simulink model "L_vs_pos_tgt"  (R2021b)
settings: Solver=ode1  StartTime=0.0  StopTime=inf  FixedStep=1e-3  RelTol=1e-3  EnableMultiTasking=on
InitFcn:
  | voltage_gain = 1;
  | current_gain = 0.5*0.1;
libraries: speedgoatlib_IO102 x3, speedgoatlib_IO301 x2, slrealtimeutilitieslib x1, slrealtimeiplib x1
settings Model: sg_rtwmakecfg_data=_sglibc_  SimulationMode=external  Creator=tcraddoc  LastModifiedBy=wasynczu
settings SolverCC: ConcurrentTasks=on  AlgebraicLoopSolver=TrustRegion  PositivePriorityOrder=on
settings DataIOCC: SaveFormat=StructureWithTime  ReturnWorkspaceOutputs=off
settings OptimizationCC: BlockReduction=off  OptimizeBlockIOStorage=off  BufferReuse=off  GlobalBufferReuse=off  ExpressionFolding=off  LocalBlockOutputs=off
settings DebuggingCC: TasksWithSamePriorityMsg=none  SFMachineParentedDataDiag=warning  ArithmeticOperatorsInVariantConditions=warning
settings HardwareCC: ProdBitPerLong=64  ProdLongLongMode=on  ProdHWDeviceType=Intel->x86-64 (Linux 64)
settings SFSimCC: SimUseLocalCustomCode=off  CustomCodeUndefinedFunction=UseInterfaceOnly
settings RTWCC: Description=Simulink Real-Time  SystemTargetFile=slrealtime.tlc  TemplateMakefile=slrealtime_default_tmf  RTWUseLocalCustomCode=off  Toolchain=Simulink Real-Time Toolchain  BuildConfiguration=Faster Runs  CodeExecutionProfiling=on  TargetLang=C++
settings CodeAppCC: StateflowObjectComments=on

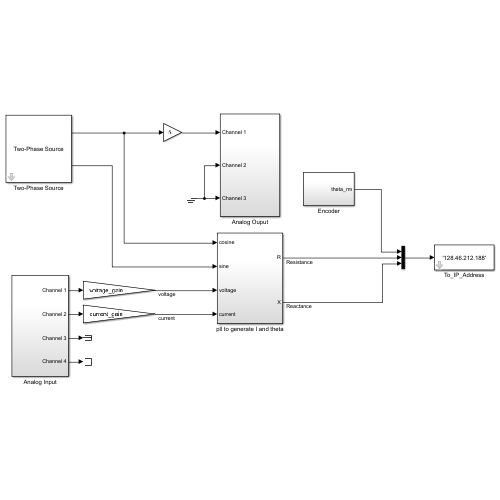
[thumbnail: Simulink's stored preview of the top-level diagram]
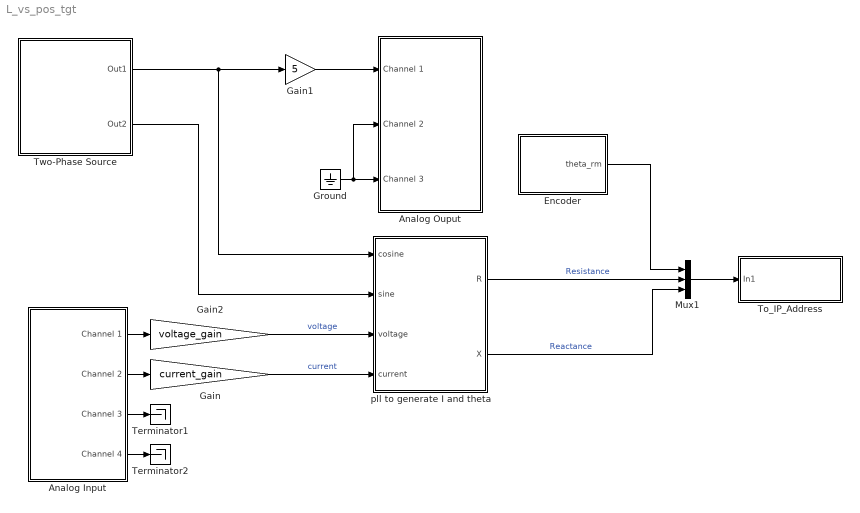
== system L_vs_pos_tgt ==
  Analog Input : Subsystem
  Analog Ouput : Subsystem
  Encoder : Subsystem
  Gain : Gain  Gain=current_gain
  Gain1 : Gain  Gain=5
  Gain2 : Gain  Gain=voltage_gain
  Ground : Ground
  Mux1 : Mux  Inputs=3
  Terminator1 : Terminator
  Terminator2 : Terminator
  To_IP_Address : Subsystem  mask{toAddress='128.46.212.188'}
      mask prompts: toAddress "To IP address"
      mask Display: disp(get_param(gcb,'toAddress'))
  Two-Phase Source : Subsystem  mask{freq=20}
      mask prompts: freq "Frequency (Hz)"
      mask Display: disp('Two-Phase Source')
  pll to generate I and theta : Subsystem
  wires:
  Two-Phase Source/1(Out1) -> pll to generate I and theta/1(cosine), Gain1/1
  Gain1/1 -> Analog Ouput/1(Channel 1)
  Ground/1 -> Analog Ouput/3(Channel 3), Analog Ouput/2(Channel 2)
  Analog Input/3(Channel 3) -> Terminator1/1
  Analog Input/4(Channel 4) -> Terminator2/1
  Two-Phase Source/2(Out2) -> pll to generate I and theta/2(sine)
  Gain/1 -> pll to generate I and theta/4(current)  "current"
  Analog Input/1(Channel 1) -> Gain2/1
  Gain2/1 -> pll to generate I and theta/3(voltage)  "voltage"
  Analog Input/2(Channel 2) -> Gain/1
  Mux1/1 -> To_IP_Address/1(In1)
  Encoder/1(theta_rm) -> Mux1/1
  pll to generate I and theta/1(R) -> Mux1/2  "Resistance"
  pll to generate I and theta/2(X) -> Mux1/3  "Reactance"

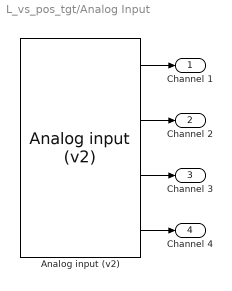
== system L_vs_pos_tgt/Analog Input ==
  "Analog input (v2) " : speedgoatlib_IO102/Analog input (v2)   id=1  channels=[1 2 3 4]  range=1  high_voltage=off  adCoupling=2  ts=1e-3  pciSlot=-1
      settings: SourceProductName=Simulink Real-Time: Speedgoat I/O Blockset
  Channel 1 : Outport
  Channel 2 : Outport  Port=2
  Channel 3 : Outport  Port=3
  Channel 4 : Outport  Port=4
  wires:
  "Analog input (v2) "/4 -> Channel 4/1
  "Analog input (v2) "/2 -> Channel 2/1
  "Analog input (v2) "/1 -> Channel 1/1
  "Analog input (v2) "/3 -> Channel 3/1

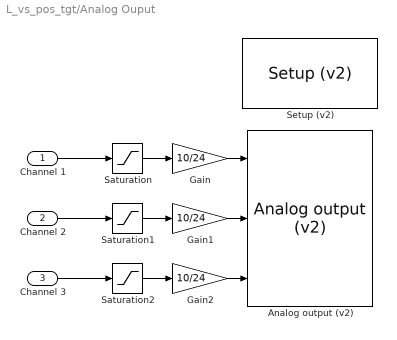
== system L_vs_pos_tgt/Analog Ouput ==
  Channel 1 : Inport
  Channel 2 : Inport  Port=2
  Channel 3 : Inport  Port=3
  "Analog output (v2) " : speedgoatlib_IO102/Analog output (v2)   id=1  channels=[1 2 3]  range=1  ts=-1  pciSlot=-1
      settings: SourceProductName=Simulink Real-Time: Speedgoat I/O Blockset
  Gain : Gain  Gain=10/24
  Gain1 : Gain  Gain=10/24
  Gain2 : Gain  Gain=10/24
  Saturation : Saturate  UpperLimit=24  LowerLimit=-24
  Saturation1 : Saturate  UpperLimit=24  LowerLimit=-24
  Saturation2 : Saturate  UpperLimit=24  LowerLimit=-24
  "Setup (v2) " : speedgoatlib_IO102/Setup (v2)   id=1  range=+-10V  cal=off  pciSlot=-1  adCoupling=Single-ended  adChannelMode=Multiple-channel (enter number of channels below)  adChannel=4  daChannel=[1,2,3]  daInitValue=[0]  daReset=[1]  DioDirectionLo=Input  DioDirectionHi=Output  doChannel=[9]  doInitValue=[0]  doReset=[1]  diChannel=[1]
      settings: SourceProductName=Simulink Real-Time: Speedgoat I/O Blockset
  wires:
  Saturation/1 -> Gain/1
  Saturation1/1 -> Gain1/1
  Saturation2/1 -> Gain2/1
  Gain1/1 -> "Analog output (v2) "/2
  Gain/1 -> "Analog output (v2) "/1
  Gain2/1 -> "Analog output (v2) "/3
  Channel 2/1 -> Saturation1/1
  Channel 3/1 -> Saturation2/1
  Channel 1/1 -> Saturation/1

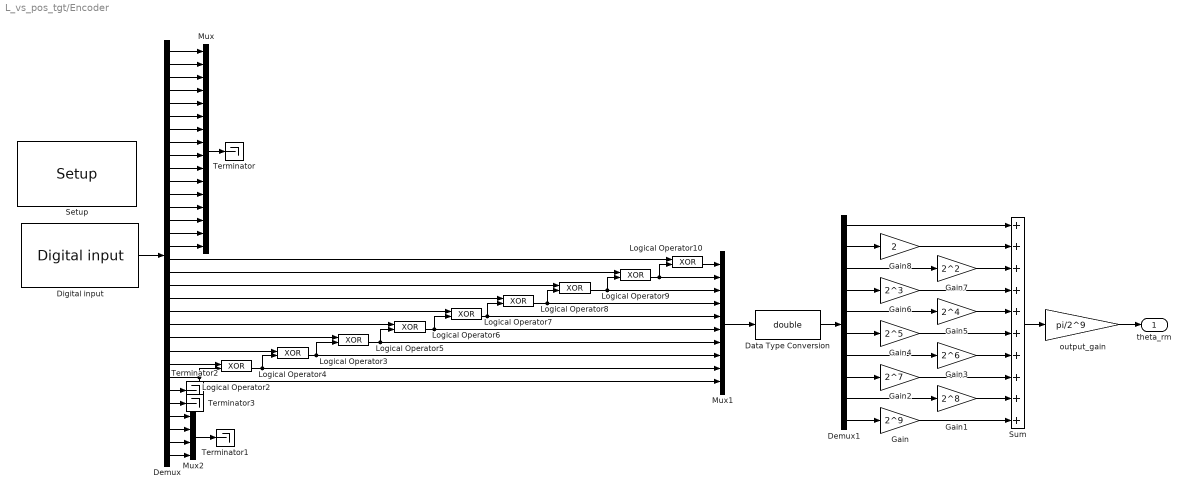
== system L_vs_pos_tgt/Encoder ==
  Data Type Conversion : DataTypeConversion  OutDataTypeStr=double
  Demux : Demux  Outputs=32
  Demux1 : Demux  Outputs=10
  Digital input : speedgoatlib_IO301/DIO/Digital input  id=1  channelGroup=Upper  portType=1 port with 32 element vector of type boolean  lowerDirection=[1,1,1,1,1,0,0,0,0,0,0,0,1,0,0,0]  upperDirection=[1,1,1,1,1,1,1,1,0,0,0,0,0,0,0,0]  ts=1e-3  pciSlot=-1
      settings: SourceProductName=Simulink Real-Time: Speedgoat I/O Blockset
  Gain : Gain  Gain=2^9
  Gain1 : Gain  Gain=2^8
  Gain2 : Gain  Gain=2^7
  Gain3 : Gain  Gain=2^6
  Gain4 : Gain  Gain=2^5
  Gain5 : Gain  Gain=2^4
  Gain6 : Gain  Gain=2^3
  Gain7 : Gain  Gain=2^2
  Gain8 : Gain  Gain=2
  Logical Operator{2..10} (9 alike) : Logic  Operator=XOR  AllPortsSameDT=off  OutDataTypeStr=boolean
  Mux : Mux  Inputs=16
  Mux1 : Mux  Inputs=10
  Mux2 : Mux
  Setup : speedgoatlib_IO301/Setup/Setup  group=Module setup  id=1  device_id=1  fpga1=speedgoat_IO301_default  pciSlot=-1  lowerDirection=[1, 1, 1, 1, 1, 0, 0, 0, 0, 0, 0, 0, 1, 0, 0, 0]  lowerReset=[1]  lowerValue=[0]  upperDirection=[1, 1, 1, 1, 1, 1, 1, 1, 0, 0, 0, 0, 0, 0, 0, 0]  upperReset=[1]  upperValue=[0]
      settings: SourceProductName=Simulink Real-Time: Speedgoat I/O Blockset
  Sum : Sum  Inputs=++++++++++
  Terminator{,1..3} (4 alike) : Terminator
  output_gain : Gain  Gain=pi/2^9
  theta_rm : Outport
  wires:
  Demux/27 -> Terminator2/1
  Demux/28 -> Terminator3/1
  Demux/26 -> Logical Operator2/2, Mux1/10
  Demux/25 -> Logical Operator2/1
  Demux/24 -> Logical Operator4/1
  Demux/23 -> Logical Operator3/1
  Demux/22 -> Logical Operator5/1
  Demux/21 -> Logical Operator6/1
  Demux/20 -> Logical Operator7/1
  Demux/19 -> Logical Operator8/1
  Demux/18 -> Logical Operator9/1
  Demux/17 -> Logical Operator10/1
  Demux1/1 -> Sum/1
  Gain8/1 -> Sum/2
  Demux1/2 -> Gain8/1
  Gain7/1 -> Sum/3
  Gain5/1 -> Sum/5
  Demux1/3 -> Gain7/1
  Gain6/1 -> Sum/4
  Demux1/4 -> Gain6/1
  Demux1/5 -> Gain5/1
  Gain4/1 -> Sum/6
  Demux1/6 -> Gain4/1
  Gain3/1 -> Sum/7
  Demux1/7 -> Gain3/1
  Gain2/1 -> Sum/8
  Demux1/8 -> Gain2/1
  Demux1/9 -> Gain1/1
  Gain1/1 -> Sum/9
  Gain/1 -> Sum/10
  Demux1/10 -> Gain/1
  Logical Operator2/1 -> Mux1/9, Logical Operator4/2
  Logical Operator4/1 -> Logical Operator3/2, Mux1/8
  Logical Operator3/1 -> Logical Operator5/2, Mux1/7
  Logical Operator5/1 -> Logical Operator6/2, Mux1/6
  Logical Operator6/1 -> Logical Operator7/2, Mux1/5
  Logical Operator7/1 -> Logical Operator8/2, Mux1/4
  Logical Operator8/1 -> Logical Operator9/2, Mux1/3
  Logical Operator10/1 -> Mux1/1
  Logical Operator9/1 -> Mux1/2, Logical Operator10/2
  output_gain/1 -> theta_rm/1
  Sum/1 -> output_gain/1
  Data Type Conversion/1 -> Demux1/1
  Mux1/1 -> Data Type Conversion/1
  Demux/32 -> Mux2/4
  Demux/31 -> Mux2/3
  Demux/30 -> Mux2/2
  Demux/29 -> Mux2/1
  Mux2/1 -> Terminator1/1
  Mux/1 -> Terminator/1
  Demux/16 -> Mux/16
  Demux/15 -> Mux/15
  Demux/14 -> Mux/14
  Demux/13 -> Mux/13
  Demux/12 -> Mux/12
  Demux/11 -> Mux/11
  Demux/10 -> Mux/10
  Demux/9 -> Mux/9
  Demux/8 -> Mux/8
  Demux/7 -> Mux/7
  Demux/6 -> Mux/6
  Demux/5 -> Mux/5
  Demux/4 -> Mux/4
  Demux/3 -> Mux/3
  Demux/2 -> Mux/2
  Demux/1 -> Mux/1
  Digital input/1 -> Demux/1

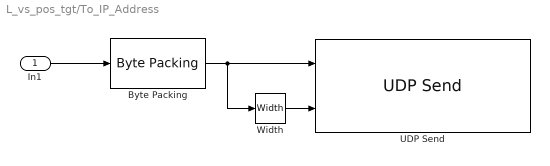
== system L_vs_pos_tgt/To_IP_Address ==
  In1 : Inport
  Byte Packing : slrealtimeutilitieslib/Byte Packing  MaskPackedDataType=uint8  MaskUnpackedDataTypes={['double']}  MaskAlignment=1
  UDP Send : slrealtimeiplib/UDP Send  useHostTargetConn=on  toAddress=toAddress  toPort=34  sampleTime=-1
      settings: SourceProductBaseCode=XP
  Width : Width
  wires:
  In1/1 -> Byte Packing/1
  Byte Packing/1 -> Width/1, UDP Send/1
  Width/1 -> UDP Send/2

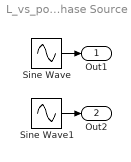
== system L_vs_pos_tgt/Two-Phase Source ==
  Sine Wave : Sin  Frequency=2*pi*freq  Phase=pi/2  SampleTime=0
  Sine Wave1 : Sin  Frequency=2*pi*freq  SampleTime=0
  Out1 : Outport
  Out2 : Outport  Port=2
  wires:
  Sine Wave/1 -> Out1/1
  Sine Wave1/1 -> Out2/1

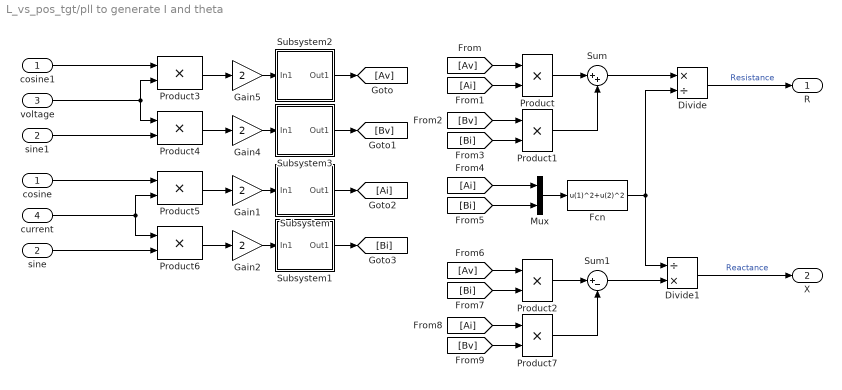
== system L_vs_pos_tgt/pll to generate I and theta ==
  cosine : Inport
  sine : Inport  Port=2
  voltage : Inport  Port=3
  current : Inport  Port=4
  Divide : Product  Inputs=*/
  Divide1 : Product  Inputs=/*
  Fcn : Fcn  Expr=u(1)^2+u(2)^2
  Gain{1..2,4..5} (4 alike) : Gain  Gain=2  SaturateOnIntegerOverflow=on  OutDataTypeStr=Inherit: Same as input  ParamDataTypeStr=Inherit: Same as input
  Mux : Mux  Inputs=2
  Product{,1..2,7} (4 alike) : Product
  Product{3..6} (4 alike) : Product  InputSameDT=on  SaturateOnIntegerOverflow=on  OutDataTypeStr=Inherit: Same as first input
  Subsystem : Subsystem  mask{T=0.05}
      mask prompts: T "averaging window"
      mask Display: disp('maf')
  Subsystem1 : Subsystem  mask{T=0.05}
      mask prompts: T "averaging window"
      mask Display: disp('maf')
  Subsystem2 : Subsystem  mask{T=1/20}
      mask prompts: T "averaging window"
      mask Display: disp('maf')
  Subsystem3 : Subsystem  mask{T=0.05}
      mask prompts: T "averaging window"
      mask Display: disp('maf')
  Sum : Sum  Inputs=|++
  Sum1 : Sum  Inputs=|+-
  cosine1 : InportShadow
  sine1 : InportShadow  Port=2
  R : Outport
  X : Outport  Port=2
  wires:
  Gain2/1 -> Subsystem1/1(In1)
  Gain1/1 -> Subsystem/1(In1)
  Product3/1 -> Gain5/1
  Gain5/1 -> Subsystem2/1(In1)
  Gain4/1 -> Subsystem3/1(In1)
  Product4/1 -> Gain4/1
  sine/1 -> Product6/2
  cosine/1 -> Product5/1
  current/1 -> Product6/1, Product5/2
  Product5/1 -> Gain1/1
  Product6/1 -> Gain2/1
  sine1/1 -> Product4/2
  cosine1/1 -> Product3/1
  voltage/1 -> Product3/2, Product4/1
  Subsystem2/1(Out1) -> [Av]
  Subsystem3/1(Out1) -> [Bv]
  Subsystem/1(Out1) -> [Ai]
  Subsystem1/1(Out1) -> [Bi]
  [Av] -> Product/1
  [Ai] -> Product/2
  [Bv] -> Product1/1
  [Bi] -> Product1/2
  Product/1 -> Sum/1
  Product1/1 -> Sum/2
  Sum/1 -> Divide/1
  Mux/1 -> Fcn/1
  [Ai] -> Mux/1
  [Bi] -> Mux/2
  Fcn/1 -> Divide1/1, Divide/2
  [Av] -> Product2/1
  [Bi] -> Product2/2
  [Ai] -> Product7/1
  [Bv] -> Product7/2
  Product2/1 -> Sum1/1
  Product7/1 -> Sum1/2
  Sum1/1 -> Divide1/2
  Divide/1 -> R/1  "Resistance"
  Divide1/1 -> X/1  "Reactance"

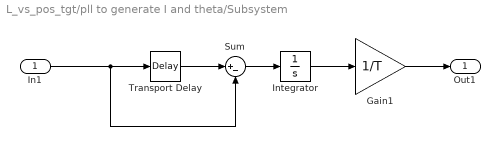
== system L_vs_pos_tgt/pll to generate I and theta/Subsystem ==
  In1 : Inport
  Gain1 : Gain  Gain=1/T  SaturateOnIntegerOverflow=on  OutDataTypeStr=Inherit: Same as input  ParamDataTypeStr=Inherit: Same as input
  Integrator : Integrator
  Sum : Sum  Inputs=|+-  InputSameDT=on  SaturateOnIntegerOverflow=on  OutDataTypeStr=Inherit: Same as first input
  Transport Delay : TransportDelay  DelayTime=T  FixedBuffer=on
  Out1 : Outport
  wires:
  Transport Delay/1 -> Sum/1
  In1/1 -> Transport Delay/1, Sum/2
  Sum/1 -> Integrator/1
  Integrator/1 -> Gain1/1
  Gain1/1 -> Out1/1

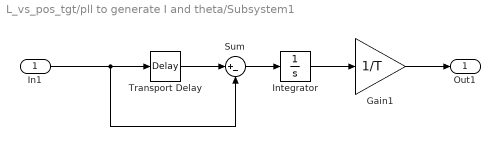
== system L_vs_pos_tgt/pll to generate I and theta/Subsystem1 ==
  In1 : Inport
  Gain1 : Gain  Gain=1/T  SaturateOnIntegerOverflow=on  OutDataTypeStr=Inherit: Same as input  ParamDataTypeStr=Inherit: Same as input
  Integrator : Integrator
  Sum : Sum  Inputs=|+-  InputSameDT=on  SaturateOnIntegerOverflow=on  OutDataTypeStr=Inherit: Same as first input
  Transport Delay : TransportDelay  DelayTime=T  FixedBuffer=on
  Out1 : Outport
  wires:
  Transport Delay/1 -> Sum/1
  In1/1 -> Transport Delay/1, Sum/2
  Sum/1 -> Integrator/1
  Integrator/1 -> Gain1/1
  Gain1/1 -> Out1/1

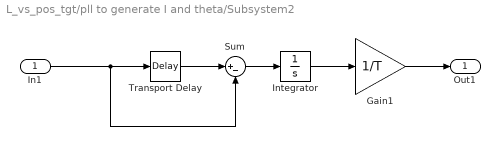
== system L_vs_pos_tgt/pll to generate I and theta/Subsystem2 ==
  In1 : Inport
  Gain1 : Gain  Gain=1/T  SaturateOnIntegerOverflow=on  OutDataTypeStr=Inherit: Same as input  ParamDataTypeStr=Inherit: Same as input
  Integrator : Integrator
  Sum : Sum  Inputs=|+-  InputSameDT=on  SaturateOnIntegerOverflow=on  OutDataTypeStr=Inherit: Same as first input
  Transport Delay : TransportDelay  DelayTime=T  FixedBuffer=on
  Out1 : Outport
  wires:
  Gain1/1 -> Out1/1
  Integrator/1 -> Gain1/1
  Sum/1 -> Integrator/1
  In1/1 -> Sum/2, Transport Delay/1
  Transport Delay/1 -> Sum/1

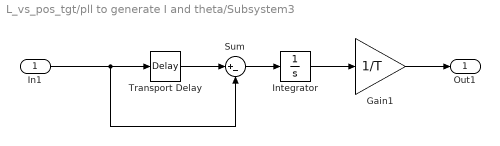
== system L_vs_pos_tgt/pll to generate I and theta/Subsystem3 ==
  In1 : Inport
  Gain1 : Gain  Gain=1/T  SaturateOnIntegerOverflow=on  OutDataTypeStr=Inherit: Same as input  ParamDataTypeStr=Inherit: Same as input
  Integrator : Integrator
  Sum : Sum  Inputs=|+-  InputSameDT=on  SaturateOnIntegerOverflow=on  OutDataTypeStr=Inherit: Same as first input
  Transport Delay : TransportDelay  DelayTime=T  FixedBuffer=on
  Out1 : Outport
  wires:
  Transport Delay/1 -> Sum/1
  In1/1 -> Transport Delay/1, Sum/2
  Sum/1 -> Integrator/1
  Integrator/1 -> Gain1/1
  Gain1/1 -> Out1/1
